simulink model "Robot_Model"  (R2022a)
settings: Solver=VariableStepAuto  StartTime=0.0  StopTime=20.0  RelTol=1e-3
values from neighbouring files (symbols this model uses):
  m = 2.5    [variables.m]
  r = 0.15    [variables.m]
undefined symbols (not defined in the file or in its folder): magnitude
libraries: simulink x1
settings Model: Creator=Bastien C  LastModifiedBy=Bastien C

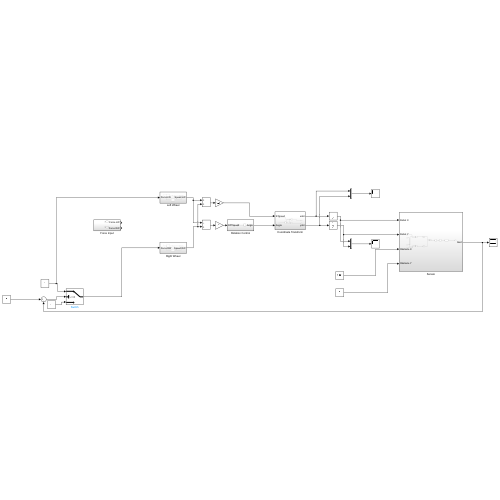
[thumbnail: Simulink's stored preview of the top-level diagram]
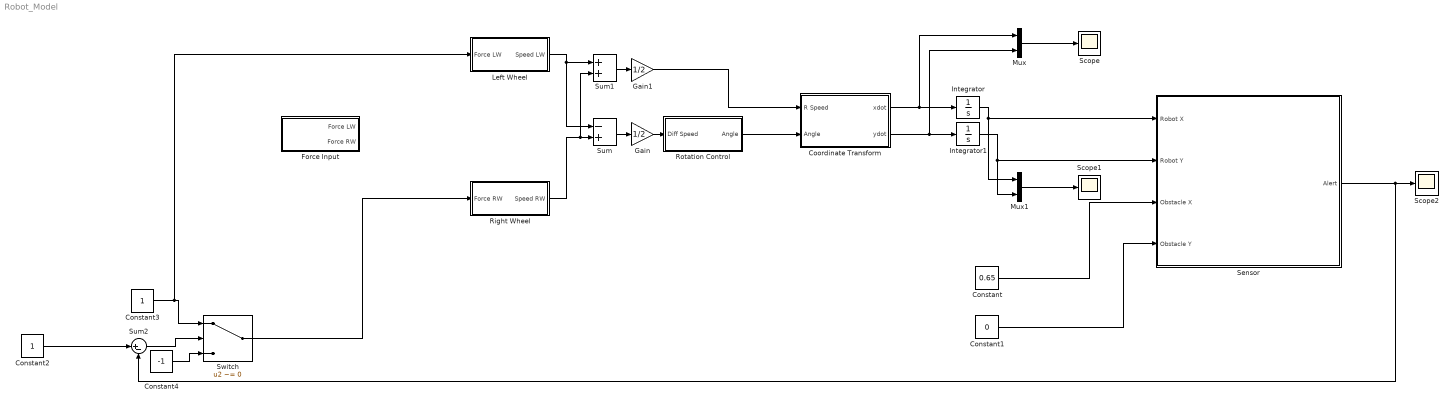
== system Robot_Model ==
  Constant : Constant  Value=0.65
  Constant1 : Constant  Value=0
  Constant2 : Constant
  Constant3 : Constant
  Constant4 : Constant  Value=-1
  Coordinate Transform : Subsystem
  Force Input : Subsystem
  Gain : Gain  Gain=1/2
  Gain1 : Gain  Gain=1/2
  Integrator : Integrator
  Integrator1 : Integrator
  Left Wheel : Subsystem
  Mux : Mux  Inputs=2
  Mux1 : Mux  Inputs=2
  Right Wheel : Subsystem
  Rotation Control : Subsystem
  Scope : Scope
  Scope1 : Scope
  Scope2 : Scope
  Sensor : Subsystem
  Sum : Sum  Inputs=-+
  Sum1 : Sum
  Sum2 : Sum  Inputs=|+-
  Switch : Switch  Criteria=u2 ~= 0  SaturateOnIntegerOverflow=off  InputSameDT=off
  wires:
  Left Wheel/1(Speed LW) -> Sum1/1, Sum/1
  Right Wheel/1(Speed RW) -> Sum1/2, Sum/2
  Sum/1 -> Gain/1
  Gain/1 -> Rotation Control/1(Diff Speed)
  Rotation Control/1(Angle) -> Coordinate Transform/2(Angle)
  Coordinate Transform/1(xdot) -> Mux/1, Integrator/1
  Coordinate Transform/2(ydot) -> Mux/2, Integrator1/1
  Sum1/1 -> Gain1/1
  Gain1/1 -> Coordinate Transform/1(R Speed)
  Mux/1 -> Scope/1
  Mux1/1 -> Scope1/1
  Integrator/1 -> Mux1/1, Sensor/1(Robot X)
  Integrator1/1 -> Sensor/2(Robot Y), Mux1/2
  Constant/1 -> Sensor/3(Obstacle X)
  Constant1/1 -> Sensor/4(Obstacle Y)
  Sensor/1(Alert) -> Sum2/2, Scope2/1
  Constant2/1 -> Sum2/1
  Sum2/1 -> Switch/2
  Constant3/1 -> Left Wheel/1(Force LW), Switch/1
  Constant4/1 -> Switch/3
  Switch/1 -> Right Wheel/1(Force RW)

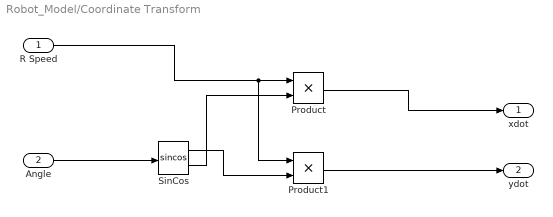
== system Robot_Model/Coordinate Transform ==
  R Speed : Inport
  Angle : Inport  Port=2
  Product : Product
  Product1 : Product
  SinCos : Trigonometry  Operator=sincos
  xdot : Outport
  ydot : Outport  Port=2
  wires:
  R Speed/1 -> Product1/1, Product/1
  Product/1 -> xdot/1
  Product1/1 -> ydot/1
  Angle/1 -> SinCos/1
  SinCos/1 -> Product1/2
  SinCos/2 -> Product/2

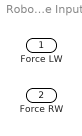
== system Robot_Model/Force Input ==
  Force LW : Outport
  Force RW : Outport  Port=2

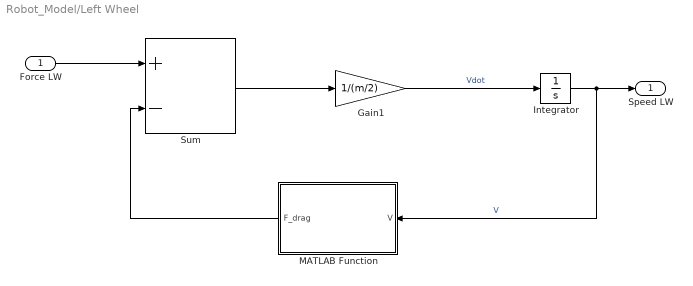
== system Robot_Model/Left Wheel ==
  Force LW : Inport
  Gain1 : Gain  Gain=1/(m/2)
  Integrator : Integrator
  MATLAB Function : MATLAB Function  TreatAsAtomicUnit=on
  Sum : Sum  Inputs=+-
  Speed LW : Outport
  wires:
  Force LW/1 -> Sum/1
  Sum/1 -> Gain1/1
  Integrator/1 -> Speed LW/1, MATLAB Function/1(V)  "V"
  Gain1/1 -> Integrator/1  "Vdot"
  MATLAB Function/1(F_drag) -> Sum/2

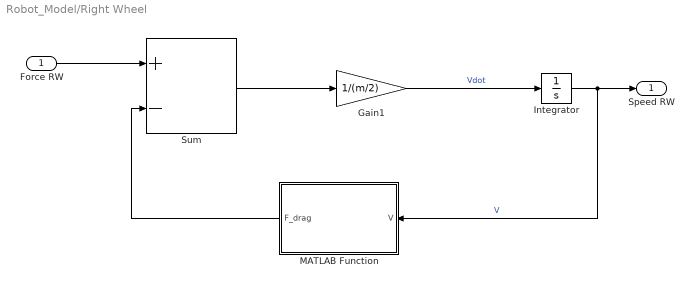
== system Robot_Model/Right Wheel ==
  Force RW : Inport
  Gain1 : Gain  Gain=1/(m/2)
  Integrator : Integrator
  MATLAB Function : MATLAB Function  TreatAsAtomicUnit=on
  Sum : Sum  Inputs=+-
  Speed RW : Outport
  wires:
  Integrator/1 -> Speed RW/1, MATLAB Function/1(V)  "V"
  Force RW/1 -> Sum/1
  Sum/1 -> Gain1/1
  Gain1/1 -> Integrator/1  "Vdot"
  MATLAB Function/1(F_drag) -> Sum/2

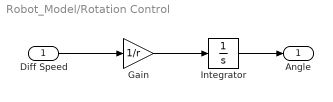
== system Robot_Model/Rotation Control ==
  Diff Speed : Inport
  Gain : Gain  Gain=1/r
  Integrator : Integrator
  Angle : Outport
  wires:
  Diff Speed/1 -> Gain/1
  Integrator/1 -> Angle/1
  Gain/1 -> Integrator/1

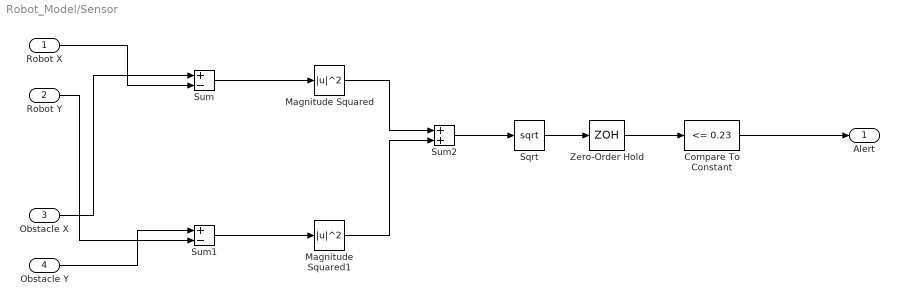
== system Robot_Model/Sensor ==
  Robot X : Inport
  Robot Y : Inport  Port=2
  Obstacle X : Inport  Port=3
  Obstacle Y : Inport  Port=4
  Compare To Constant : simulink/Logic and Bit Operations/Compare To Constant  relop=<=  const=0.23  OutDataTypeStr=boolean
  Magnitude Squared : Math  Operator=magnitude^2
  Magnitude Squared1 : Math  Operator=magnitude^2
  Sqrt : Sqrt
  Sum : Sum  Inputs=+-
  Sum1 : Sum  Inputs=+-
  Sum2 : Sum
  Zero-Order Hold : ZeroOrderHold  SampleTime=0.25
  Alert : Outport
  wires:
  Robot X/1 -> Sum/2
  Obstacle X/1 -> Sum/1
  Robot Y/1 -> Sum1/2
  Obstacle Y/1 -> Sum1/1
  Sum1/1 -> Magnitude Squared1/1
  Sum/1 -> Magnitude Squared/1
  Magnitude Squared/1 -> Sum2/1
  Magnitude Squared1/1 -> Sum2/2
  Sum2/1 -> Sqrt/1
  Compare To Constant/1 -> Alert/1
  Sqrt/1 -> Zero-Order Hold/1
  Zero-Order Hold/1 -> Compare To Constant/1

== matlab function Robot_Model/Left Wheel/MATLAB Function ==
  data: V input; F_drag output; k_drag parameter
function F_drag = get_Fdrag(V, k_drag)

F_drag = k_drag * V * abs(V);

== matlab function Robot_Model/Right Wheel/MATLAB Function ==
  data: V input; F_drag output; k_drag parameter
function F_drag = get_Fdrag(V, k_drag)

F_drag = k_drag * V * abs(V);
